simulink model "class_d"  (R2024b)
settings: Solver=VariableStepAuto  StartTime=0.0  StopTime=5e-3  MaxStep=1e-8  RelTol=1e-9
undefined symbols (not defined in the file): gaussian
libraries: simulink x2
settings Model: SimulationMode=rapid-accelerator  Creator=Aaron  LastModifiedBy=Aaron
settings SolverCC: ShapePreserveControl=EnableAll  ZeroCrossAlgorithm=Adaptive

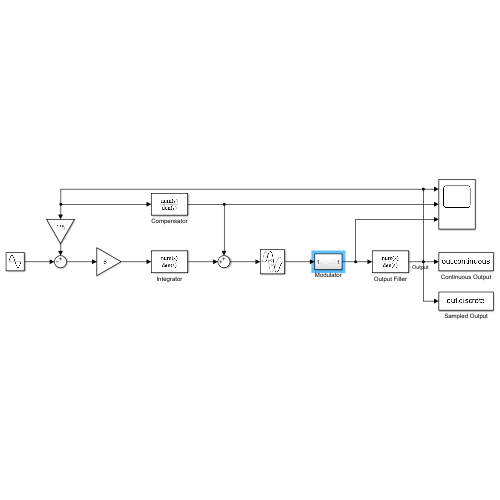
[thumbnail: Simulink's stored preview of the top-level diagram]
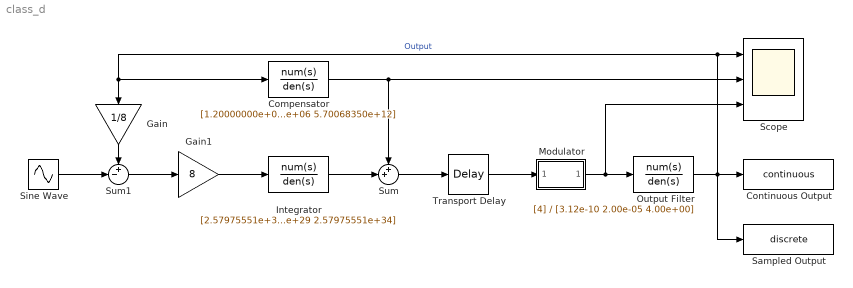
== system class_d ==
  Compensator : TransferFcn  Numerator=[1.20000000e+00 3.01592895e+06 1.89496405e+12]  Denominator=[1.00000000e+00 4.77522083e+06 5.70068350e+12]
  Continuous Output : ToWorkspace  VariableName=continuous  SaveFormat=Structure With Time  SampleTime=-1
  Gain : Gain  Gain=1/8
  Gain1 : Gain  Gain=8
  Integrator : TransferFcn  Numerator=[2.57975551e+34]  Denominator=[1.00000000e+00 4.17465908e+06 6.64489620e+12 5.12635184e+18 2.02101886e+24 3.75508392e+29 2.57975551e+34]
  Modulator : Subsystem
  Output Filter : TransferFcn  Numerator=[4]  Denominator=[3.12e-10 2.00e-05 4.00e+00]
  Sampled Output : ToWorkspace  VariableName=discrete  SampleTime=-1
  Scope : Scope  NumInputPorts=3
  Sine Wave : Sin  Amplitude=4  Frequency=2*pi*1e3  SampleTime=0
  Sum : Sum  Inputs=++|
  Sum1 : Sum  Inputs=+-|
  Transport Delay : TransportDelay  DelayTime=120e-9
  wires:
  Transport Delay/1 -> Modulator/1(Input)
  Modulator/1(Output) -> Scope/3, Output Filter/1
  Sum/1 -> Transport Delay/1
  Integrator/1 -> Sum/2
  Compensator/1 -> Sum/1, Scope/2
  Sine Wave/1 -> Sum1/2
  Sum1/1 -> Gain1/1
  Gain/1 -> Sum1/1
  Output Filter/1 -> Sampled Output/1, Continuous Output/1, Compensator/1, Gain/1, Scope/1  "Output"
  Gain1/1 -> Integrator/1

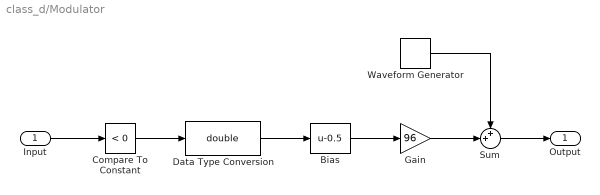
== system class_d/Modulator ==
  Input : Inport
  Bias : Bias  Bias=-0.5  SaturateOnIntegerOverflow=off
  Compare To Constant : simulink/Logic and Bit Operations/Compare To Constant  relop=<  const=0  OutDataTypeStr=uint8
  Data Type Conversion : DataTypeConversion  OutDataTypeStr=double  SaturateOnIntegerOverflow=off  RndMeth=Floor
  Gain : Gain  Gain=96
  Sum : Sum  Inputs=++|
  Waveform Generator : simulink/Sources/Waveform Generator  OutMin=[]  OutMax=[]  OutDataTypeStr=double  SelectedSignal=1  Signals=gaussian()  BlockNames=MultiportSwitch_63dad018c2994e4  SampleTime=0.1
  Output : Outport
  wires:
  Input/1 -> Compare To Constant/1
  Data Type Conversion/1 -> Bias/1
  Compare To Constant/1 -> Data Type Conversion/1
  Bias/1 -> Gain/1
  Gain/1 -> Sum/2
  Sum/1 -> Output/1
  Waveform Generator/1 -> Sum/1
